simulink subsystem "Vel_Ruedas_PWM"  (R2024b)
settings: Solver=VariableStepAuto  StartTime=0.0  StopTime=10.0  RelTol=1e-3
settings Model: Creator=Chenfu  LastModifiedBy=Chenfu

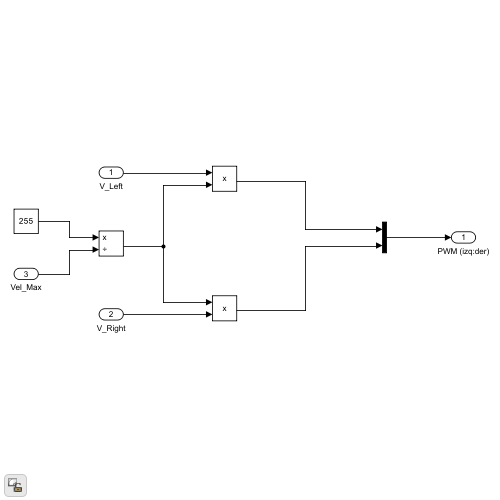
[thumbnail: Simulink's stored preview of the top-level diagram]
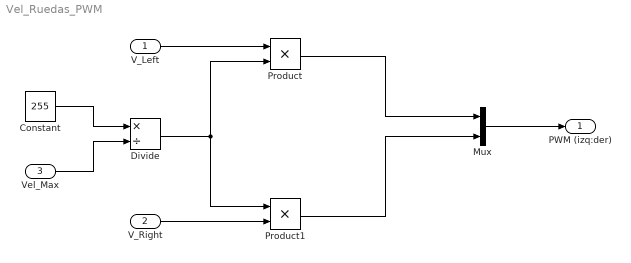
== system Vel_Ruedas_PWM ==
  V_Left : Inport
  V_Right : Inport  Port=2
  Vel_Max : Inport  Port=3
  Constant : Constant  Value=255
  Divide : Product  Inputs=*/
  Mux : Mux  Inputs=2
  Product : Product
  Product1 : Product
  PWM (izq:der) : Outport
  wires:
  Mux/1 -> PWM (izq:der)/1
  V_Right/1 -> Product1/2
  V_Left/1 -> Product/1
  Divide/1 -> Product1/1, Product/2
  Constant/1 -> Divide/1
  Vel_Max/1 -> Divide/2
  Product/1 -> Mux/1
  Product1/1 -> Mux/2
